simulink model "lab5_E2_b"  (R2020a)
settings: Solver=FixedStepAuto  StartTime=0.0  StopTime=20  FixedStep=0.01  RelTol=1e-3
values from neighbouring files (symbols this model uses):
  p = path    [pplane8.m]
undefined symbols (not defined in the file or in its folder): K_p, M, T_d, T_i
settings Model: Creator=bruno  LastModifiedBy=bruno

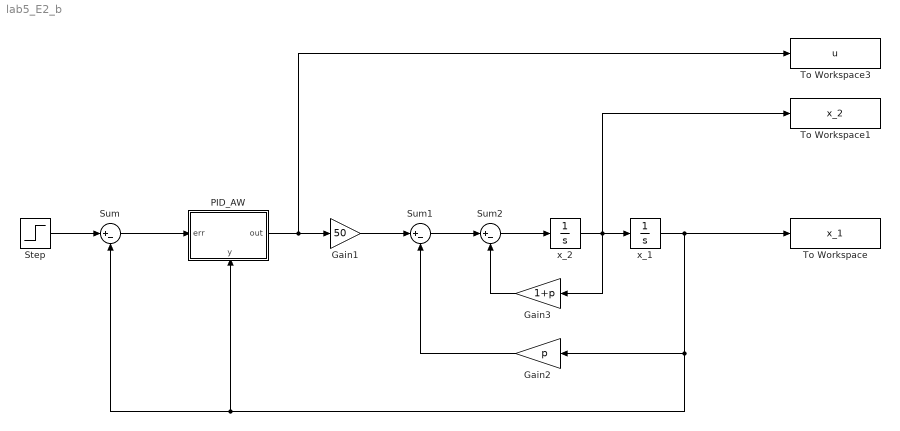
== system lab5_E2_b ==
  Gain1 : Gain  Gain=50
  Gain2 : Gain  Gain=p
  Gain3 : Gain  Gain=1+p
  PID_AW : Subsystem
      settings: PortSchema="{\"entries\":[{\"content\":{\"sides\":[{\"content\":{\"connectorIds\":[\"In1\"]},\"type\":\"ConnectorPlacement.EquallySpacedRectSide\",\"uuid\":\"c0bc5389-6fa5-4218-970b-51ad75fb133e\"},{\"content\":{\"connectorIds\":[\"Out1\"],\"side\":\"RIGHT\"},\"type\":\"ConnectorPlacement.EquallySpacedRectSide\",\"uuid\":\"2b714c0f-b3df-4a82-a715-7a42ae590ae1\"},{\"content\":{\"connectorIds\":[],\"side\":\"TOP\"},\"type\":\"ConnectorPlacement.EquallySpacedRectSide\",\"uuid\":\"9a703cbf-0350-48a9-81e3-8ef42d98dc5c\"},{\"content\":{\"connectorIds\":[\"In2\"],\"side\":\"BOTTOM\"},\"type\":\"ConnectorPlacement.EquallySpacedRectSide\",\"uuid\":\"349667ab-6eb2-4393-9583-ac386b6b3734\"}]},\"type\":\"ConnectorPlacement.EquallySpacedConnector\",\"uuid\":\"2ba20ed9-8bba-4569-b243-9718a616a2fa\"}],\"packageUris\":[\"http://schema.mathworks.com/mf0/Connector/19700101\"],\"version\":\"1.0\"}"
  Step : Step  Time=0  SampleTime=0
  Sum : Sum  Inputs=|+-
  Sum1 : Sum  Inputs=|+-
  Sum2 : Sum  Inputs=|+-
  To Workspace : ToWorkspace  VariableName=x_1  SaveFormat=Timeseries  SampleTime=-1
  To Workspace1 : ToWorkspace  VariableName=x_2  SaveFormat=Timeseries  SampleTime=-1
  To Workspace3 : ToWorkspace  VariableName=u  SaveFormat=Timeseries  SampleTime=-1
  x_1 : Integrator
  x_2 : Integrator
  wires:
  Step/1 -> Sum/1
  Gain1/1 -> Sum1/1
  Sum1/1 -> Sum2/1
  Sum2/1 -> x_2/1
  x_2/1 -> To Workspace1/1, Gain3/1, x_1/1
  x_1/1 -> PID_AW/2(y), Sum/2, Gain2/1, To Workspace/1
  Gain2/1 -> Sum1/2
  Gain3/1 -> Sum2/2
  Sum/1 -> PID_AW/1(err)
  PID_AW/1(out) -> To Workspace3/1, Gain1/1

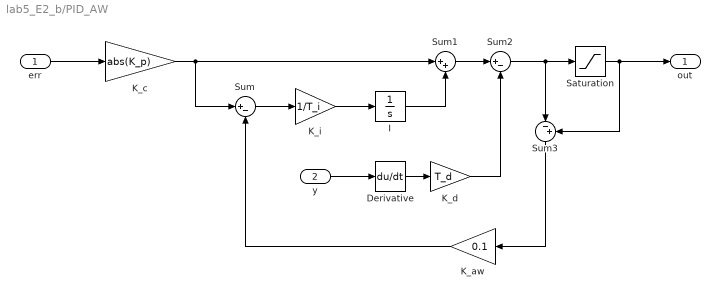
== system lab5_E2_b/PID_AW ==
  err : Inport
  y : Inport  Port=2
  Derivative : Derivative
  I : Integrator
  K_aw : Gain  Gain=0.1
  K_c : Gain  Gain=abs(K_p)
  K_d : Gain  Gain=T_d
  K_i : Gain  Gain=1/T_i
  Saturation : Saturate  UpperLimit=M  LowerLimit=-M
  Sum : Sum  Inputs=|+-
  Sum1 : Sum  Inputs=|++
  Sum2 : Sum  Inputs=|+-
  Sum3 : Sum  Inputs=|-+
  out : Outport
  wires:
  K_aw/1 -> Sum/2
  K_d/1 -> Sum2/2
  Sum1/1 -> Sum2/1
  Sum3/1 -> K_aw/1
  K_i/1 -> I/1
  Sum/1 -> K_i/1
  Saturation/1 -> out/1, Sum3/2
  Sum2/1 -> Sum3/1, Saturation/1
  Derivative/1 -> K_d/1
  y/1 -> Derivative/1
  I/1 -> Sum1/2
  err/1 -> K_c/1
  K_c/1 -> Sum1/1, Sum/1
